simulink model "z4_discPI"  (R2020a)
settings: Solver=ode45  StartTime=0.0  StopTime=50  RelTol=1e-3
values from neighbouring files (symbols this model uses):
  ki = 0.48    [spraw4.m]
  kp = 3    [spraw4.m]
  Ts = 0.1    [spraw4.m]
undefined symbols (not defined in the file or in its folder): d_denominator, d_numerator, DiscIntNeverNeededParam
settings Model: Creator=admin  LastModifiedBy=admin

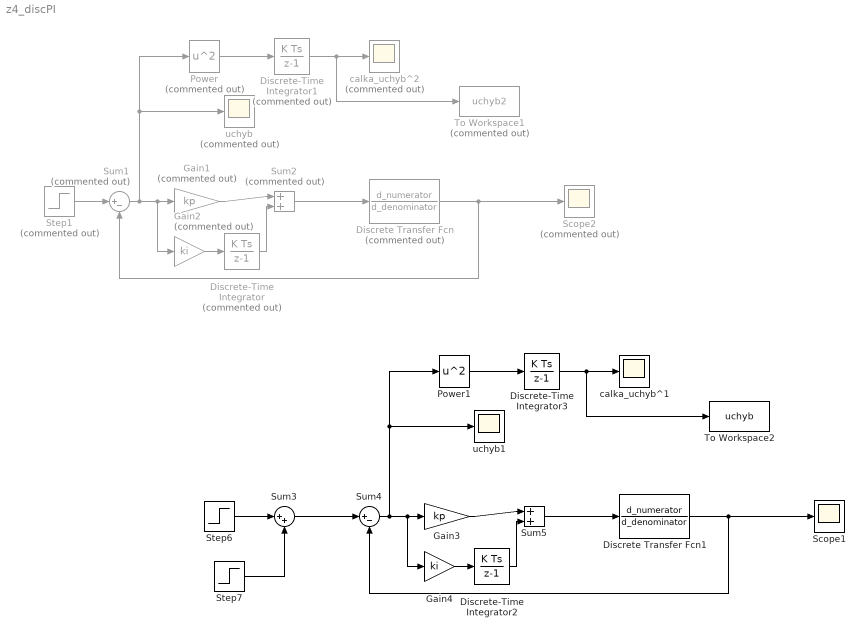
== system z4_discPI ==
  Discrete Transfer Fcn : DiscreteTransferFcn  Commented=on  Numerator=d_numerator  Denominator=d_denominator
  Discrete Transfer Fcn1 : DiscreteTransferFcn  Numerator=d_numerator  Denominator=d_denominator
  Discrete-Time Integrator : DiscreteIntegrator  Commented=on  SampleTime=Ts  ICPrevOutput=DiscIntNeverNeededParam  ICPrevScaledInput=DiscIntNeverNeededParam
  Discrete-Time Integrator1 : DiscreteIntegrator  Commented=on  SampleTime=Ts  ICPrevOutput=DiscIntNeverNeededParam  ICPrevScaledInput=DiscIntNeverNeededParam
  Discrete-Time Integrator2 : DiscreteIntegrator  SampleTime=Ts  ICPrevOutput=DiscIntNeverNeededParam  ICPrevScaledInput=DiscIntNeverNeededParam
  Discrete-Time Integrator3 : DiscreteIntegrator  SampleTime=Ts  ICPrevOutput=DiscIntNeverNeededParam  ICPrevScaledInput=DiscIntNeverNeededParam
  Gain1 : Gain  Commented=on  Gain=kp
  Gain2 : Gain  Commented=on  Gain=ki
  Gain3 : Gain  Gain=kp
  Gain4 : Gain  Gain=ki
  Power : Math  Commented=on  Operator=square  SaturateOnIntegerOverflow=on
  Power1 : Math  Operator=square  SaturateOnIntegerOverflow=on
  Scope1 : Scope
  Scope2 : Scope  Commented=on
  Step1 : Step  Commented=on  SampleTime=0
  Step6 : Step  After=100000  SampleTime=0
  Step7 : Step  Time=1.0001  After=-100000  SampleTime=0
  Sum1 : Sum  Commented=on  Inputs=|+-
  Sum2 : Sum  Commented=on  Inputs=|++
  Sum3 : Sum  Inputs=|++
  Sum4 : Sum  Inputs=|+-
  Sum5 : Sum  Inputs=|++
  To Workspace1 : ToWorkspace  Commented=on  VariableName=uchyb2  SaveFormat=Timeseries  SampleTime=Ts
  To Workspace2 : ToWorkspace  VariableName=uchyb  SaveFormat=Timeseries  SampleTime=Ts
  calka_uchyb^1 : Scope
  calka_uchyb^2 : Scope  Commented=on
  uchyb : Scope  Commented=on
  uchyb1 : Scope
  wires:
  Power/1 -> Discrete-Time Integrator1/1
  Sum1/1 -> Power/1, uchyb/1, Gain2/1, Gain1/1
  Discrete Transfer Fcn/1 -> Sum1/2, Scope2/1
  Discrete-Time Integrator/1 -> Sum2/2
  Sum2/1 -> Discrete Transfer Fcn/1
  Discrete-Time Integrator1/1 -> To Workspace1/1, calka_uchyb^2/1
  Gain1/1 -> Sum2/1
  Step1/1 -> Sum1/1
  Gain2/1 -> Discrete-Time Integrator/1
  Gain4/1 -> Discrete-Time Integrator2/1
  Discrete-Time Integrator3/1 -> To Workspace2/1, calka_uchyb^1/1
  Sum3/1 -> Sum4/1
  Discrete-Time Integrator2/1 -> Sum5/2
  Power1/1 -> Discrete-Time Integrator3/1
  Sum5/1 -> Discrete Transfer Fcn1/1
  Sum4/1 -> Power1/1, uchyb1/1, Gain4/1, Gain3/1
  Discrete Transfer Fcn1/1 -> Sum4/2, Scope1/1
  Gain3/1 -> Sum5/1
  Step7/1 -> Sum3/2
  Step6/1 -> Sum3/1
